simulink model "verification_zoom"  (R2015b)
settings: Solver=VariableStepAuto  StartTime=0.0  StopTime=inf  RelTol=1e-3
libraries: neural x20, visionstatistics x1, visionconversions x1, visiongeotforms x1, visionsinks x1
(part 2 of 5)

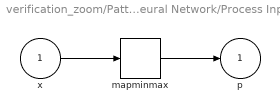
== system verification_zoom/Pattern Recognition Neural Network/Process Input 1 ==
  x : Inport  PortDimensions=4800
      mask Display: e = 0.06;c1 = [120 230 180]/255;c2 = ([120 230 180]+0)/(256+128);c3 = ([120 230 180]+128)/(256+128);patch([0 1 1 0],[0 0 1 1],c1);patch([0 1 1 1-e 1-e 0+e],[0 0 1 1-e 0+e 0+e],c2);patch([0 0 1 1-e 0+e 0+e],[0 1 1 1-e 1-e 0+e],c3);plot([0 1 1 0 0],[0 0 1 1 0]);
  mapminmax : neural/Processing Functions/mapminmax  xmin=[0.058823529411764705;0.050980392156862744;0.062745098039215685;0.11372549019607843;0.13725490196078433;0.10588235294117647;0.078431372549019607;0.094117647058823528;0.12156862745098039;0.11764705882352941;0.12549019607843137;0.19215686274509805;0.10980392156862745;0.15686274509803921;0.25098039215686274;0.25490196078431371;0.30980392156862746;0.17254901960784313;0.094117647058823528;0.074509803921568626;0.11372549019607843;0.070588235294117646;0.058823529411764705;0.058823529411764705;0.066666666666666666;0.023529411764705882;0.043137254901960784;0.070588235294117646;0.070588235294117646;0.082352941176470587;0.12941176470588237;0.18431372549019609;0.2627450980392157;0.20000000000000001;0.10588235294117647;0.16078431372549021;0.25490196078431371;0.31764705882352939;0.38039215686274508;0.31764705882352939;0.066666666666666666;0.054901960784313725;0.074509803921568626;0.11372549019607843;0.11372549019607843;0.094117647058823528;0.10196078431372549;0.12156862745098039;0.10980392156862745;0.10980392156862745;0.16862745098039217;0.19215686274509805;0.18431372549019609;0.16862745098039217;0.12941176470588237;0.2196078431372549;0.34901960784313724;0.17647058823529413;0.13333333333333333;0.062745098039215685;0.035294117647058823;0.050980392156862744;0.058823529411764705;0.050980392156862744;0.050980392156862744;0.043137254901960784;0.035294117647058823;0.031372549019607843;0.031372549019607843;0.043137254901960784;0.10588235294117647;0.18823529411764706;0.21176470588235294;0.26666666666666666;0.14901960784313725;0.082352941176470587;0.10588235294117647;0.12156862745098039;0.17254901960784313;0.18431372549019609;0.070588235294117646;0.050980392156862744;0.058823529411764705;0.10588235294117647;0.12941176470588237;0.18823529411764706;0.090196078431372548;0.086274509803921567;0.086274509803921567;0.090196078431372548;0.14901960784313725;0.19215686274509805;0.19215686274509805;0.27058823529411763;0.23137254901960785;0.33725490196078434;0.27058823529411763;0.16862745098039217;0.13725490196078433;0.062745098039215685;0.023529411764705882;0.019607843137254902;0.027450980392156862;0.019607843137254902;0.019607843137254902;0.031372549019607843;0.023529411764705882;0.015686274509803921;0.023529411764705882;0.043137254901960784;0.13333333333333333;0.20392156862745098;0.20000000000000001;0.30980392156862746;0.41176470588235292;0.22352941176470589;0.047058823529411764;0.031372549019607843;0.031372549019607843;0.043137254901960784;0.070588235294117646;0.058823529411764705;0.058823529411764705;0.10196078431372549;0.10588235294117647;0.11764705882352941;0.12941176470588237;0.098039215686274508;0.15686274509803921;0.12549019607843137;0.11372549019607843;0.15294117647058825;0.21176470588235294;0.24313725490196078;0.29803921568627451;0.50980392156862742;0.16078431372549021;0.15686274509803921;0.17254901960784313;0.12941176470588237;0.019607843137254902;0.011764705882352941;0.015686274509803921;0.011764705882352941;0.0078431372549019607;0.015686274509803921;0.035294117647058823;0.027450980392156862;0.019607843137254902;0.054901960784313725;0.14901960784313725;0.17647058823529413;0.18431372549019609;0.16470588235294117;0.16470588235294117;0.19215686274509805;0.078431372549019607;0.019607843137254902;0.023529411764705882;0.019607843137254902;0.050980392156862744;0.050980392156862744;0.054901960784313725;0.086274509803921567;0.14509803921568629;0.10196078431372549;0.082352941176470587;0.098039215686274508;0.15294117647058825;0.18823529411764706;0.18823529411764706;0.12941176470588237;0.12549019607843137;0.23137254901960785;0.49019607843137253;0.28235294117647058;0.094117647058823528;0.15686274509803921;0.14509803921568629;0.090196078431372548;0.011764705882352941;0.015686274509803921;0.011764705882352941;0.019607843137254902;0.015686274509803921;0.019607843137254902;0.035294117647058823;0.031372549019607843;0.039215686274509803;0.074509803921568626;0.13333333333333333;0.13333333333333333;0.13725490196078433;0.13725490196078433;0.12941176470588237 ...(+94023 chars)]  xmax=[1;1;1;1;1;1;1;1;1;1;1;1;0.99607843137254903;1;1;1;1;1;1;1;1;1;1;1;1;1;1;1;1;1;1;1;1;1;1;1;1;1;1;1;1;1;1;1;1;1;1;1;1;1;1;1;1;0.99607843137254903;1;1;0.99607843137254903;1;1;1;1;1;1;1;1;1;1;1;1;1;1;1;1;1;1;1;1;1;1;1;1;1;1;1;1;1;1;1;1;1;1;1;0.99607843137254903;0.99607843137254903;1;1;1;1;1;1;1;1;1;1;1;1;1;1;1;1;1;1;1;1;1;1;1;1;1;1;1;0.99607843137254903;1;1;1;1;1;0.99607843137254903;1;1;0.99607843137254903;1;1;1;1;1;1;1;1;1;1;1;1;1;1;1;1;1;1;1;1;1;1;1;1;1;1;1;1;1;0.99607843137254903;1;1;1;1;1;0.99607843137254903;1;1;1;1;1;1;1;1;1;1;1;1;1;1;0.99607843137254903;1;1;1;1;1;1;1;1;1;1;1;1;1;1;1;1;1;1;1;0.99607843137254903;1;1;1;0.99607843137254903;0.99607843137254903;0.99607843137254903;1;1;1;1;1;0.99607843137254903;1;0.99607843137254903;1;1;1;1;1;1;1;0.99607843137254903;1;1;1;1;1;1;1;1;1;1;1;1;1;1;1;1;0.99607843137254903;1;1;1;1;1;0.99607843137254903;1;0.99607843137254903;0.99607843137254903;0.99607843137254903;1;0.99607843137254903;0.99607843137254903;0.99607843137254903;0.99607843137254903;1;1;1;1;1;1;1;0.99607843137254903;0.99607843137254903;1;1;1;1;1;1;1;1;1;1;1;1;1;1;1;0.99607843137254903;0.99607843137254903;1;1;1;1;0.99607843137254903;1;1;0.99607843137254903;0.99607843137254903;1;0.99607843137254903;0.99607843137254903;0.99607843137254903;1;1;1;1;1;1;1;0.99607843137254903;0.99607843137254903;0.99607843137254903;0.99607843137254903;0.99607843137254903;1;1;1;1;1;1;1;1;1;1;1;1;1;0.99607843137254903;0.99607843137254903;1;1;0.99607843137254903;0.99607843137254903;0.99607843137254903;1;0.99607843137254903;0.99607843137254903;1;1;0.99607843137254903;1;0.99607843137254903;1;1;1;0.99607843137254903;0.99607843137254903;0.99607843137254903;1;1;0.99607843137254903;0.99607843137254903;0.99607843137254903;0.99607843137254903;1;1;1;1;1;1;1;1;1;1;1;1;1;0.99607843137254903;0.99607843137254903;0.99607843137254903;1;1;1;1;1;0.99607843137254903;0.99607843137254903;1;0.99607843137254903;0.99607843137254903;1;1;1;0.99607843137254903;1;0.99607843137254903;0.99607843137254903;0.99607843137254903;0.99607843137254903;0.99215686274509807;0.99215686274509807;0.99607843137254903;0.99607843137254903;0.99607843137254903;0.99607843137254903;0.99607843137254903;0.99607843137254903;0.99607843137254903;0.99607843137254903;1;1;1;1;1;1;1;1;1;1;0.99607843137254903;1;1;1;0.99607843137254903;1;1;0.99607843137254903;0.99607843137254903;0.99607843137254903;0.99607843137254903;0.99607843137254903;0.99607843137254903;1;0.99607843137254903;1;0.99607843137254903;0.99607843137254903;0.99215686274509807;0.99607843137254903;0.99607843137254903;0.9882352941176471;0.99607843137254903;0.99215686274509807;0.99607843137254903;0.99215686274509807;0.99607843137254903;0.99607843137254903;0.99607843137254903;0.99607843137254903;1;1;1;1;1;1;1;1;0.99607843137254903;0.99607843137254903;1;1;1;0.99607843137254903;1;1;0.99607843137254903;0.99607843137254903;0.99607843137254903;1;0.99607843137254903;1;0.99607843137254903;0.99607843137254903;0.99607843137254903;0.99215686274509807;0.99215686274509807;0.99607843137254903;0.99215686274509807;0.99215686274509807;0.9882352941176471;0.99215686274509807;0.9882352941176471;0.9882352941176471;0.99607843137254903;0.99607843137254903;0.99607843137254903;0.99607843137254903;0.99607843137254903;0.99607843137254903;0.99607843137254903;1;1;1;1;1;1;1;0.99607843137254903;0.99607843137254903;1;1;1;0.99607843137254903;0.99607843137254903;1;1;1;1;0.99607843137254903;0.99607843137254903;0.99607843137254903;0.99607843137254903;0.99215686274509807;0.99607843137254903;0.99215686274509807;0.99215686274509807;0.99215686274509807;0.98431372549019602;0.99215686274509807;0.9882352941176471;0.9882352941176471;0.9882352941176471;0.98431372549019602;0.9882352941176471;0.99607843137254903;0.99607843137254903;0.99607843137254903;0.99215686274509807;0.99607843137254903;1;1;1;1;1;1;1;1;1;1;1;0.99607843137254903;1;1;1;0.99607843137254903;0.99607843137254903;1;1;0.99607843137254903;1;0.99215686274509807;0.99215686274509807;0.99215686274509807;0.99215686274509807 ...(+75203 chars)]  ymin=-1  ymax=1
  p : Outport  PortDimensions=4800
      mask Display: e = 0.06;c1 = [120 230 180]/255;c2 = ([120 230 180]+0)/(256+128);c3 = ([120 230 180]+128)/(256+128);patch([0 1 1 0],[0 0 1 1],c1);patch([0 1 1 1-e 1-e 0+e],[0 0 1 1-e 0+e 0+e],c2);patch([0 0 1 1-e 0+e 0+e],[0 1 1 1-e 1-e 0+e],c3);plot([0 1 1 0 0],[0 0 1 1 0]);
  wires:
  x/1 -> mapminmax/1
  mapminmax/1 -> p/1
